simulink model "ContinousCounterAndDelayBlock"  (R2013a)
settings: Solver=ode3  StartTime=0.0  StopTime=10.0  RelTol=1e-3
libraries: simulink x1
settings Model: Creator=ajdin  LastModifiedBy=ajdin

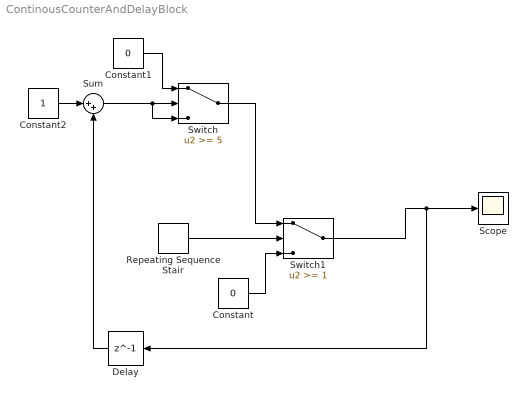
== system ContinousCounterAndDelayBlock ==
  Constant : Constant  Value=0
  Constant1 : Constant  Value=0
  Constant2 : Constant
  Delay : Delay  DelayLength=1  InitialCondition=0
  Repeating Sequence Stair : simulink/Sources/Repeating Sequence Stair  OutValues=[1 1].'  tsamp=-1  OutMin=[]  OutMax=[]  OutDataTypeStr=double  OutputDataTypeScalingMode=double  OutDataType=fixdt(0,8)  ConRadixGroup=Best Precision: Vector-wise  OutScaling=2^-12
  Scope : Scope
  Sum : Sum  Inputs=|++
  Switch : Switch  Threshold=5
  Switch1 : Switch  Threshold=1
  wires:
  Switch1/1 -> Delay/1, Scope/1
  Delay/1 -> Sum/2
  Repeating Sequence Stair/1 -> Switch1/2
  Constant/1 -> Switch1/3
  Switch/1 -> Switch1/1
  Constant1/1 -> Switch/1
  Sum/1 -> Switch/3, Switch/2
  Constant2/1 -> Sum/1
